simulink model "Simulinkproject2"  (Simulink 8.1)
settings: Solver=ode45  StartTime=0.0  StopTime=10.0  RelTol=1e-3
values from neighbouring files (symbols this model uses):
  D = 0.03    [matlabsimulink.m]    (also in matlabsimulink2.m = 3)
  I = 0    [matlabsimulink.m]    (also in matlabsimulink2.m = 35)
  P = Kp_d*D    (= 0.78)    [matlabsimulink.m]    (also in matlabsimulink2.m = 30)
undefined symbols (not defined in the file or in its folder): sigbuilder_block
libraries: cstblocks x1
settings Model: Creator=mehmetserdargurman  LastModifiedBy=Mertcan Kaya
settings DebuggingCC: FcnCallInpInsideContextMsg=EnableAllAsWarning
settings GRTTargetCC: CombineOutputUpdateFcns=on  GRTInterface=off

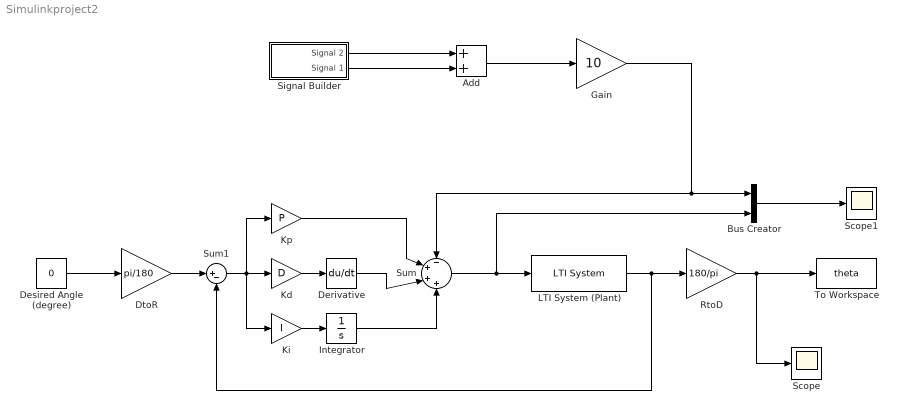
== system Simulinkproject2 ==
  Add : Sum
  Bus Creator : BusCreator  Inputs=2
  Derivative : Derivative
  Desired Angle (degree) : Constant  Value=0
  DtoR : Gain  Gain=pi/180
  Gain : Gain  Gain=10
  Integrator : Integrator
  Kd : Gain  Gain=D
  Ki : Gain  Gain=I
  Kp : Gain  Gain=P
  LTI System (Plant) : cstblocks/LTI System  sys=plant  IC=[]
  RtoD : Gain  Gain=180/pi
  Scope : Scope
  Scope1 : Scope
  Signal Builder : Subsystem  Tag=STV Subsys  LoadFcn=sigbuilder_block('load');  StartFcn=sigbuilder_block('start');  StopFcn=sigbuilder_block('stop');  ClipboardFcn=sigbuilder_block('clipboard');  mask(Sigbuilder block){}
      mask help: Create and generate interchangeable groups of signals whose waveforms are piecewise linear.
      mask init:
      | if ~strcmp(get_param(bdroot(gcbh),'SimulationStatus'),'stopped') tuvar = sigbuilder_block('maskInit'); end
      settings: CopyFcn=sigbuilder_block('copy');  DeleteFcn=sigbuilder_block('delete');  ModelCloseFcn=sigbuilder_block('modelClose');  PreSaveFcn=sigbuilder_block('preSave');  PauseFcn=sigbuilder_block('pause')  ContinueFcn=sigbuilder_block('continue')  NameChangeFcn=sigbuilder_block('namechange');  OpenFcn=sigbuilder_block('open',[196.5 85.5 550.5 427.5 ]);  CloseFcn=sigbuilder_block('close');
      mask Display: plot(0,0,100,100,[10,10,40,40,10],[80,20,20,80,80],[40,10],[50,50], [40,27,10],[65,72,56],[40,25,25,10],[28,28,43,43]);
  Sum : Sum  Inputs=-+++
  Sum1 : Sum  Inputs=|+-
  To Workspace : ToWorkspace  VariableName=theta  SampleTime=-1  SaveFormat=Structure With Time
  wires:
  Kd/1 -> Derivative/1
  Ki/1 -> Integrator/1
  Sum/1 -> LTI System (Plant)/1, Bus Creator/2
  LTI System (Plant)/1 -> RtoD/1, Sum1/2
  Sum1/1 -> Ki/1, Kp/1, Kd/1
  Desired Angle (degree)/1 -> DtoR/1
  DtoR/1 -> Sum1/1
  Integrator/1 -> Sum/4
  Derivative/1 -> Sum/3
  Kp/1 -> Sum/2
  Add/1 -> Gain/1
  Gain/1 -> Sum/1, Bus Creator/1
  Bus Creator/1 -> Scope1/1
  RtoD/1 -> To Workspace/1, Scope/1
  Signal Builder/1(Signal 2) -> Add/1
  Signal Builder/2(Signal 1) -> Add/2

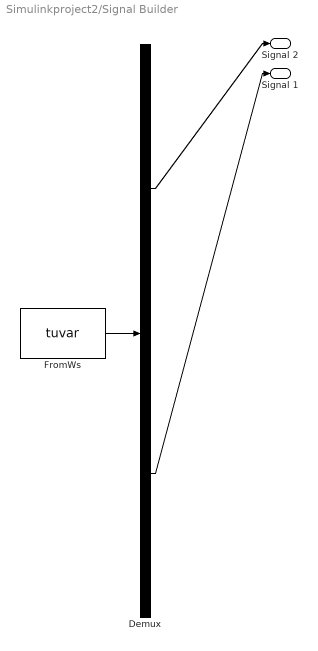
== system Simulinkproject2/Signal Builder ==
  Demux : Demux  Tag=STV Demux  Outputs=2
  FromWs : FromWorkspace  Tag=STV FromWs  VariableName=tuvar  SampleTime=0  SigBuilderData=DataTag0  VnvData=DataTag1
      SigBuilderData=|
      | common.afterFinalStr = 'Extrapolate'
      | common.sampleTime = 0
      | dataSet.timeRange = [0 10]
      | dataSet.name = 'Group 1'
      | sbobj.Groups.Name = 'Group 1'
      | sbobj.Groups.Signals(1).Name = 'Signal 2'
      | sbobj.Groups.Signals(1).XData = [0 5 5 5.2 5.2 10]
      | sbobj.Groups.Signals(1).YData = [0 0 -0.08 -0.08 0 0]
      | sbobj.Groups.Signals(2).Name = 'Signal 1'
      | sbobj.Groups.Signals(2).XData = [0 0.2 0.2 10]
      | sbobj.Groups.Signals(2).YData = [0.146 0.146 0 0]
  Signal 2 : Outport  Tag=STV Outport
  Signal 1 : Outport  Tag=STV Outport  Port=2
  wires:
  FromWs/1 -> Demux/1
  Demux/1 -> Signal 2/1
  Demux/2 -> Signal 1/1
